simulink model "PID_uGrid_changed_by_code"  (R2020a)
settings: Solver=VariableStepAuto  StartTime=0.0  StopTime=0.08  RelTol=1e-3
values from neighbouring files (symbols this model uses):
  I_pv_sp_V = 0.0662*Ir_V+0.0549    [Simulation_PID_variable_conditions.m]    (also in Simulation_variable_PID_ANN_gain_selector.m; Simulation_variable_PID_Interpolated_gain_selector.m; Simulation_variable_PID_KNN_gain_selector.m)
  Ir_V = [0 100 500 1000 500 100 0]    [Simulation_PID_variable_conditions.m]    (also in Simulation_variable_PID_ANN_gain_selector.m; Simulation_variable_PID_Interpolated_gain_selector.m; Simulation_variable_PID_KNN_gain_selector.m)
  RL_var_vec = [1 6 8 15 7 3 5]    [Simulation_PID_variable_conditions.m]    (also in Simulation_variable_PID_ANN_gain_selector.m; Simulation_variable_PID_Interpolated_gain_selector.m; Simulation_variable_PID_KNN_gain_selector.m)
  tim_vec = 0:1:6    [Simulation_PID_variable_conditions.m]    (also in Simulation_variable_PID_ANN_gain_selector.m; Simulation_variable_PID_Interpolated_gain_selector.m; Simulation_variable_PID_KNN_gain_selector.m)
undefined symbols (not defined in the file or in its folder): fmicro, Ion, Lithium
libraries: powerlib x15, simulink x3, powerlib_meascontrol x3, eeStairGenerator x3, electricdrivelib x1, re_lib x1
settings Model: Creator=Javier  LastModifiedBy=Javier

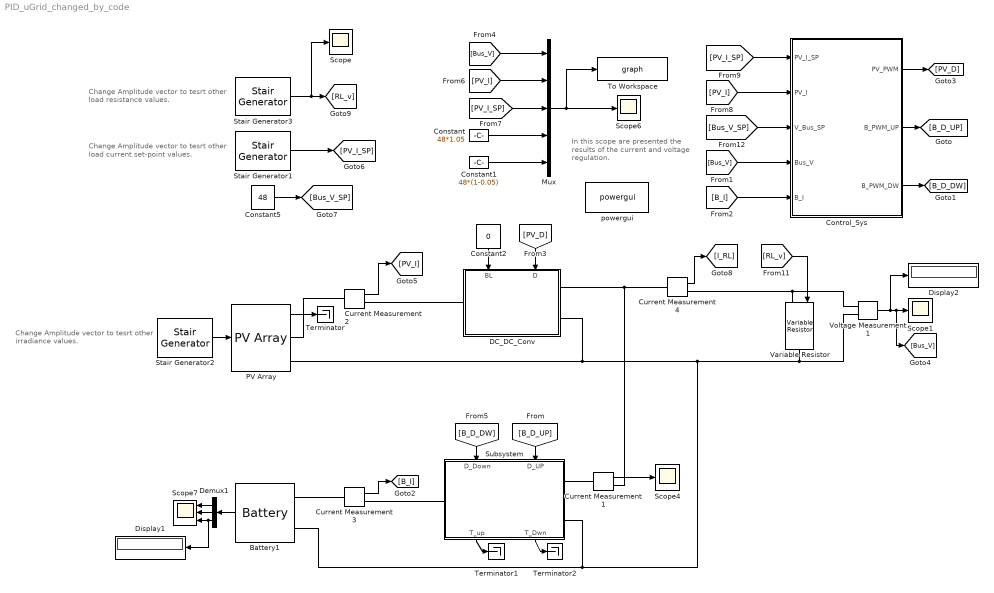
== system PID_uGrid_changed_by_code ==
  note: Change Amplitude vector to tesrt other
      | load resistance values.
  note: Change Amplitude vector to tesrt other
      | load current set-point values.
  note: Change Amplitude vector to tesrt other
      | irradiance values.
  note: In this scope are presented the
      | results of the current and voltage
      | regulation.
  Battery1 : electricdrivelib/Extra Sources/Battery  BatType=Lithium-Ion  ShowTempParam=off  ThermalPreset=no  ShowAgeParam=off  NomV=38.4  NomQ=2500  SOC=60  Batt_Tr=30  PresetModel=on  MaxQ=2500  MinV=28.8  FullV=44.6971  Dis_rate=1086.9565  R=0.0001536  Normal_OP=2260.8696  expZone="[41.48682      122.8261]"  current=[6.5 13 32.5]  Units=Time  Tci=20  NomT=20  T2=-30  MaxQ2=4.8  FullV2=7.1  Normal_OP2=5.655  expZone2="[6.58           1]"  Rca=0.6  ti=2000  Dp=0  Neq0=0  Tsim=1e6  Ta1=25  Qeol=5.4*0.9  Reol=0.013333*1.2  Char_age=[2.3478, 3]  Dis_age=[2.3478, 10]  N1=1500  N2=10500  N3=1000  N4=1400  Ta2=45  N5=950
  Constant : Constant  Value=48*1.05
  Constant1 : Constant  Value=48*(1-0.05)
  Constant2 : Constant  Value=0
  Constant5 : Constant  Value=48
  Control_Sys : Subsystem
  Current Measurement{1..4} (4 alike) : powerlib/Measurements/Current Measurement  PhasorSimulation=off  OutputType=Complex  PSBequivalent=0
  DC_DC_Conv : Subsystem
      settings: PortSchema="{\"entries\":[{\"content\":{\"sides\":[{\"content\":{\"connectorIds\":[\"LConn1\"]},\"type\":\"ConnectorPlacement.EquallySpacedRectSide\",\"uuid\":\"00f7090b-60ae-413e-b809-f771630d6751\"},{\"content\":{\"connectorIds\":[\"RConn1\",\"RConn2\"],\"side\":\"RIGHT\"},\"type\":\"ConnectorPlacement.EquallySpacedRectSide\",\"uuid\":\"f0025ab7-a9d8-466a-8e23-704d013948c1\"},{\"content\":{\"connectorIds\":[\"In1\",\"In2\"],\"side\":\"TOP\"},\"type\":\"ConnectorPlacement.EquallySpacedRectSide\",\"uuid\":\"5a345099-75bf-400d-9bb3-22f689fa92ef\"}]},\"type\":\"ConnectorPlacement.EquallySpacedConnector\",\"uuid\":\"2e1b2c5d-1adb-4779-83d3-3c40793dd951\"}],\"packageUris\":[\"http://schema.mathworks.com/mf0/Connector/19700101\"],\"version\":\"1.0\"}"
  Demux1 : Demux  Outputs=3
  Display1 : Display
  Display2 : Display
  Mux : Mux  Inputs=5
  PV Array : re_lib/Solar/PV Array  Npar=7  Nser=1  PlotType=array @ 1000 W/m2 & specified temperatures  S_vec="[ 1000  500  100 ]"  Temp_C_vec="[ 45 25  ]"  ModuleName=LG Electronics LG300N1W-G3  PlotWhenSelected=off  Pm=302.72  Ncell=60  Voc=39.5  Isc=10.05  Vm=32  Im=9.46  beta_Voc_pc=-0.3  alpha_Isc_pc=0.03  beta_Voc=-0.1185  alpha_Isc=0.003015  IL=10.0926  I0=3.3235e-11  nI=0.96984  Rsh=212.8143  Rs=0.31448  RobustModel=on  RobustCellTemperature=25  BAL=on  Tc=1e-7  Tfilter=1e-8
  Scope{,1,4,6} (4 alike) : Scope
  Scope7 : Scope  NumInputPorts=3
  Stair Generator1 : eeStairGenerator/Stair Generator  LabelModeActiveChoice=Discrete  TimeInput=[tim_vec]*0.01  AmplitudeInput=[I_pv_sp_V]  SampleTime=1/(1000e3)  RepeatPattern=off  OutDataTypeStr=double
      settings: SourceProductBaseCode=PS
  Stair Generator2 : eeStairGenerator/Stair Generator  LabelModeActiveChoice=Discrete  TimeInput=[tim_vec]*0.01  AmplitudeInput=[Ir_V]  SampleTime=1/(1000e3)  RepeatPattern=off  OutDataTypeStr=double
      settings: SourceProductBaseCode=PS
  Stair Generator3 : eeStairGenerator/Stair Generator  LabelModeActiveChoice=Discrete  TimeInput=[tim_vec]*0.01  AmplitudeInput=[RL_var_vec]  SampleTime=1/(1000e3)  RepeatPattern=off  OutDataTypeStr=double
      settings: SourceProductBaseCode=PS
  Subsystem : Subsystem
      settings: PortSchema="{\"entries\":[{\"content\":{\"sides\":[{\"content\":{\"connectorIds\":[\"LConn1\"]},\"type\":\"ConnectorPlacement.EquallySpacedRectSide\",\"uuid\":\"a9530ab3-8980-4dba-8483-d408c1c24a59\"},{\"content\":{\"connectorIds\":[\"RConn1\",\"RConn2\"],\"side\":\"RIGHT\"},\"type\":\"ConnectorPlacement.EquallySpacedRectSide\",\"uuid\":\"f691113d-6eb3-43ec-a6a4-3d8fb6884df6\"},{\"content\":{\"connectorIds\":[\"In1\",\"In2\"],\"side\":\"TOP\"},\"type\":\"ConnectorPlacement.EquallySpacedRectSide\",\"uuid\":\"a9eb11b6-05d7-4dbc-be9d-a17fd8550bb3\"},{\"content\":{\"connectorIds\":[\"Out1\",\"Out2\"],\"side\":\"BOTTOM\"},\"type\":\"ConnectorPlacement.EquallySpacedRectSide\",\"uuid\":\"90c7147c-e357-433a-9063-3b2a71587c45\"}]},\"type\":\"ConnectorPlacement.EquallySpacedConnector\",\"uuid\":\"b290d60f-d8ab-41f4-904b-2a909013e95d\"}],\"packageUris\":[\"http://schema.mathworks.com/mf0/Connector/19700101\"],\"version\":\"1.0\"}"
  Terminator : Terminator
  Terminator1 : Terminator
  Terminator2 : Terminator
  To Workspace : ToWorkspace  VariableName=graph  SaveFormat=Timeseries  SampleTime=-1
  Variable Resistor : powerlib/Elements/Variable Resistor  Rabsmin=1e-3
      settings: SourceProductBaseCode=PS
  Voltage Measurement1 : powerlib/Measurements/Voltage Measurement  PhasorSimulation=off  OutputType=Complex  PSBequivalent=0
  powergui : powerlib/powergui  Priority=1  SimulationMode=Discrete  SampleTime=1/(1000e3)  frequency=60  Iterations=50  frequencyindice=0  Pbase=100e6  ErrMax=1e-4  UnitsV=kV  UnitsW=MW  buscounter=0  FunctionMessages=off  echomessages=off  EnableUseOfTLC=off  CurrentSourceSwitches=off  DisableSnubberDevices=off  DisableRonSwitches=off  DisableVfSwitches=off  DisplayEquations=off  AutomaticDiscreteSolvers=off  SolverType=Tustin/Backward Euler (TBE)  Interpol=off  ExternalGateDelay=off  methode=off  Ts=100  x0status=blocks  SPID=on  SwTol=0  HookPort=off  NonlinearTolerance=1e-4  nMaxIteration=100  ContinueOnMaxIteration=off  RestoreLinks=warning  ResistiveCurrentMeasurement=off  Frange=[0:2:500]  Ylog=off  Xlog=on  ShowGrid=off  save=off  variable=ZData  structure=0  ZoomFFT=off  StartTime=0.0  cycles=1  DisplayStyle=1  fundamental=60  FreqAxis=off  MaxFrequency=1000  frequencyindicesteady=1  RmsSteady=1  display=off
  wires:
  Current Measurement1/1 -> Scope4/1
  Constant1/1 -> Mux/5
  Stair Generator2/1 -> PV Array/1
  Subsystem/1(T_up) -> Terminator1/1
  Subsystem/2(T_Dwn) -> Terminator2/1
  [B_D_UP] -> Subsystem/2(D_UP)
  [PV_I_SP] -> Control_Sys/1(PV_I_SP)
  [Bus_V] -> Mux/1
  [B_D_DW] -> Subsystem/1(D_Down)
  [PV_I] -> Control_Sys/2(PV_I)
  [Bus_V_SP] -> Control_Sys/3(V_Bus_SP)
  Constant5/1 -> [Bus_V_SP]
  Control_Sys/2(B_PWM_UP) -> [B_D_UP]
  [Bus_V] -> Control_Sys/4(Bus_V)
  PV Array/1 -> Terminator/1
  Current Measurement4/1 -> [I_RL]
  Battery1/1 -> Demux1/1
  Current Measurement3/1 -> [B_I]
  Constant2/1 -> DC_DC_Conv/1(BL)
  Control_Sys/3(B_PWM_DW) -> [B_D_DW]
  [PV_I] -> Mux/2
  Current Measurement2/1 -> [PV_I]
  Stair Generator3/1 -> Scope/1, [RL_v]
  Demux1/2 -> Scope7/2
  Control_Sys/1(PV_PWM) -> [PV_D]
  [B_I] -> Control_Sys/5(B_I)
  Voltage Measurement1/1 -> [Bus_V], Scope1/1, Display2/1
  [PV_I_SP] -> Mux/3
  Stair Generator1/1 -> [PV_I_SP]
  [RL_v] -> Variable Resistor/1
  Demux1/3 -> Display1/1, Scope7/3
  Demux1/1 -> Scope7/1
  Constant/1 -> Mux/4
  [PV_D] -> DC_DC_Conv/2(D)
  Mux/1 -> To Workspace/1, Scope6/1
  connections:
  DC_DC_Conv/RConn1 -- Current Measurement1/RConn1 -- Current Measurement4/LConn1
  Battery1/LConn2 -- Variable Resistor/RConn1 -- Voltage Measurement1/LConn2 -- DC_DC_Conv/RConn2 -- PV Array/RConn2 -- Subsystem/RConn2
  Voltage Measurement1/LConn1 -- Current Measurement4/RConn1 -- Variable Resistor/LConn1
  Current Measurement3/RConn1 -- Subsystem/LConn1
  Current Measurement2/RConn1 -- DC_DC_Conv/LConn1
  Current Measurement3/LConn1 -- Battery1/LConn1
  Current Measurement1/LConn1 -- Subsystem/RConn1
  Current Measurement2/LConn1 -- PV Array/RConn1

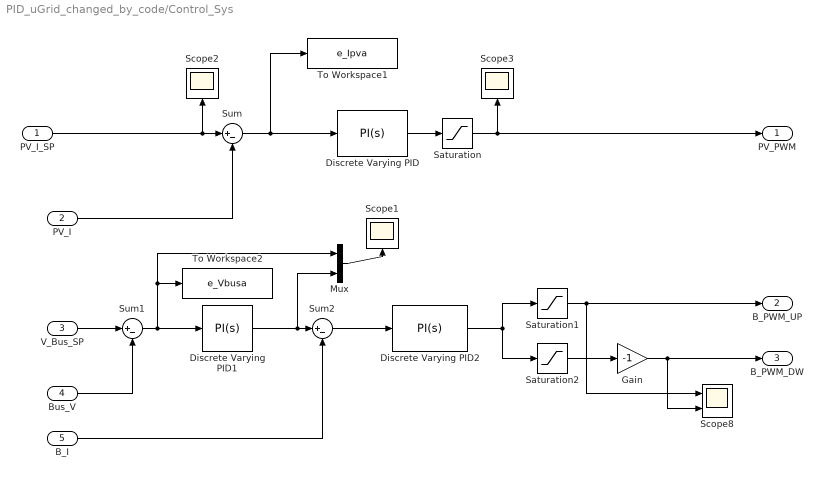
== system PID_uGrid_changed_by_code/Control_Sys ==
  PV_I_SP : Inport
  PV_I : Inport  Port=2
  V_Bus_SP : Inport  Port=3
  Bus_V : Inport  Port=4
  B_I : Inport  Port=5
  Discrete Varying PID : simulink/Continuous/PID Controller  Controller=PI  Form=Parallel  TimeDomain=Continuous-time  UseExternalTs=off  SampleTime=1/fmicro  IntegratorMethod=Forward Euler  FilterMethod=Forward Euler  ControllerParametersSource=internal  P=480.2696  I=467.6542  D=0  UseFilter=on  N=100  TunerSelectOption=Transfer Function Based (PID Tuner App)  InitialConditionSource=internal  InitialConditionForIntegrator=0  InitialConditionForFilter=0  DifferentiatorICPrevScaledInput=0  ExternalReset=none  TrackingMode=off  Kt=1  LimitOutput=on  UpperSaturationLimit=1  LowerSaturationLimit=-1  LinearizeAsGain=on  AntiWindupMode=none  Kb=1  POutMin=[]  POutMax=[]  IOutMin=[]  IOutMax=[]  DOutMin=[]  DOutMax=[]  NOutMin=[]  NOutMax=[]  SumOutMin=[]  SumOutMax=[]  SaturationOutMin=[]  SaturationOutMax=[]  PParamMin=[]  PParamMax=[]  IParamMin=[]  IParamMax=[]  DParamMin=[]  DParamMax=[]  NParamMin=[]  NParamMax=[]  KbParamMin=[]  KbParamMax=[]  KtParamMin=[]  KtParamMax=[]  KbOutMin=[]  KbOutMax=[]  KtOutMin=[]  KtOutMax=[]  IntegratorOutMin=[]  IntegratorOutMax=[]  FilterOutMin=[]  FilterOutMax=[]  SumI1OutMin=[]  SumI1OutMax=[]  SumI2OutMin=[]  SumI2OutMax=[]  SumI3OutMin=[]  SumI3OutMax=[]  SumI4OutMin=[]  SumI4OutMax=[]  SumDOutMin=[]  SumDOutMax=[]  DifferentiatorOutMin=[]  DifferentiatorOutMax=[]  FilterDiffOutCoefMin=[]  FilterDiffOutCoefMax=[]  ReciprocalOutMin=[]  ReciprocalOutMax=[]  SumDenOutMin=[]  SumDenOutMax=[]  SumNumOutMin=[]  SumNumOutMax=[]  DivideOutMin=[]  DivideOutMax=[]  UdiffTsProdOutMin=[]  UdiffTsProdOutMax=[]  NTsProdOutMin=[]  NTsProdOutMax=[]  UintegralTsProdOutMin=[]  UintegralTsProdOutMax=[]  UngainTsProdOutMin=[]  UngainTsProdOutMax=[]  IntegratorContinuousStateAttributes=''  IntegratorStateMustResolveToSignalObject=off  IntegratorRTWStateStorageClass=Auto  FilterContinuousStateAttributes=''  FilterStateMustResolveToSignalObject=off  FilterRTWStateStorageClass=Auto  ParallelPVariant=InternalParameters  IdealPVariant=Disabled  IVariant=InternalParameters  DVariant=Disabled  IntegratorVariant=Continuous  SatVariant=Enabled  AWVariant=Passthrough  PCopyVariant=Disabled  TRVariant=Disabled  FdbkBlocksVariant=Forward  IdealPFdbkVariant=Disabled  SatFdbkVariant=Disabled  DerivativeFilterVariant=Disabled  NVariant=Disabled  NCopyVariant=Disabled_SignalSpec  FilterICVariant=Disabled  IntegratorICVariant=InternalICs  ExternalResetVariant=Disabled  TRSumVariant=Passthrough  SumFdbkVariant=Disabled  SumVariant=Sum_PI  TsampFilterVariant=InternalTs  TsampNgainVariant=Passthrough  TsampIntegralVariant=Passthrough
  Discrete Varying PID1 : simulink/Continuous/PID Controller  Controller=PI  Form=Parallel  TimeDomain=Continuous-time  UseExternalTs=off  SampleTime=1/fmicro  IntegratorMethod=Forward Euler  FilterMethod=Forward Euler  ControllerParametersSource=internal  P=92.8314  I=4.166  D=0  UseFilter=on  N=100  TunerSelectOption=Transfer Function Based (PID Tuner App)  InitialConditionSource=internal  InitialConditionForIntegrator=0  InitialConditionForFilter=0  DifferentiatorICPrevScaledInput=0  ExternalReset=none  TrackingMode=off  Kt=1  LimitOutput=off  UpperSaturationLimit=500  LowerSaturationLimit=-500  LinearizeAsGain=on  AntiWindupMode=none  Kb=1  POutMin=[]  POutMax=[]  IOutMin=[]  IOutMax=[]  DOutMin=[]  DOutMax=[]  NOutMin=[]  NOutMax=[]  SumOutMin=[]  SumOutMax=[]  SaturationOutMin=[]  SaturationOutMax=[]  PParamMin=[]  PParamMax=[]  IParamMin=[]  IParamMax=[]  DParamMin=[]  DParamMax=[]  NParamMin=[]  NParamMax=[]  KbParamMin=[]  KbParamMax=[]  KtParamMin=[]  KtParamMax=[]  KbOutMin=[]  KbOutMax=[]  KtOutMin=[]  KtOutMax=[]  IntegratorOutMin=[]  IntegratorOutMax=[]  FilterOutMin=[]  FilterOutMax=[]  SumI1OutMin=[]  SumI1OutMax=[]  SumI2OutMin=[]  SumI2OutMax=[]  SumI3OutMin=[]  SumI3OutMax=[]  SumI4OutMin=[]  SumI4OutMax=[]  SumDOutMin=[]  SumDOutMax=[]  DifferentiatorOutMin=[]  DifferentiatorOutMax=[]  FilterDiffOutCoefMin=[]  FilterDiffOutCoefMax=[]  ReciprocalOutMin=[]  ReciprocalOutMax=[]  SumDenOutMin=[]  SumDenOutMax=[]  SumNumOutMin=[]  SumNumOutMax=[]  DivideOutMin=[]  DivideOutMax=[]  UdiffTsProdOutMin=[]  UdiffTsProdOutMax=[]  NTsProdOutMin=[]  NTsProdOutMax=[]  UintegralTsProdOutMin=[]  UintegralTsProdOutMax=[]  UngainTsProdOutMin=[]  UngainTsProdOutMax=[]  IntegratorContinuousStateAttributes=''  IntegratorStateMustResolveToSignalObject=off  IntegratorRTWStateStorageClass=Auto  FilterContinuousStateAttributes=''  FilterStateMustResolveToSignalObject=off  FilterRTWStateStorageClass=Auto  ParallelPVariant=InternalParameters  IdealPVariant=Disabled  IVariant=InternalParameters  DVariant=Disabled  IntegratorVariant=Continuous  SatVariant=Disabled  AWVariant=Passthrough  PCopyVariant=Disabled  TRVariant=Disabled  FdbkBlocksVariant=Forward  IdealPFdbkVariant=Disabled  SatFdbkVariant=Disabled  DerivativeFilterVariant=Disabled  NVariant=Disabled  NCopyVariant=Disabled_SignalSpec  FilterICVariant=Disabled  IntegratorICVariant=InternalICs  ExternalResetVariant=Disabled  TRSumVariant=Passthrough  SumFdbkVariant=Disabled  SumVariant=Sum_PI  TsampFilterVariant=InternalTs  TsampNgainVariant=Passthrough  TsampIntegralVariant=Passthrough
  Discrete Varying PID2 : simulink/Continuous/PID Controller  Controller=PI  Form=Parallel  TimeDomain=Continuous-time  UseExternalTs=off  SampleTime=1/fmicro  IntegratorMethod=Forward Euler  FilterMethod=Forward Euler  ControllerParametersSource=internal  P=0.01  I=36.8058  D=0  UseFilter=on  N=100  TunerSelectOption=Transfer Function Based (PID Tuner App)  InitialConditionSource=internal  InitialConditionForIntegrator=0  InitialConditionForFilter=0  DifferentiatorICPrevScaledInput=0  ExternalReset=none  TrackingMode=off  Kt=1  LimitOutput=on  UpperSaturationLimit=1  LowerSaturationLimit=-1  LinearizeAsGain=on  AntiWindupMode=none  Kb=1  POutMin=[]  POutMax=[]  IOutMin=[]  IOutMax=[]  DOutMin=[]  DOutMax=[]  NOutMin=[]  NOutMax=[]  SumOutMin=[]  SumOutMax=[]  SaturationOutMin=[]  SaturationOutMax=[]  PParamMin=[]  PParamMax=[]  IParamMin=[]  IParamMax=[]  DParamMin=[]  DParamMax=[]  NParamMin=[]  NParamMax=[]  KbParamMin=[]  KbParamMax=[]  KtParamMin=[]  KtParamMax=[]  KbOutMin=[]  KbOutMax=[]  KtOutMin=[]  KtOutMax=[]  IntegratorOutMin=[]  IntegratorOutMax=[]  FilterOutMin=[]  FilterOutMax=[]  SumI1OutMin=[]  SumI1OutMax=[]  SumI2OutMin=[]  SumI2OutMax=[]  SumI3OutMin=[]  SumI3OutMax=[]  SumI4OutMin=[]  SumI4OutMax=[]  SumDOutMin=[]  SumDOutMax=[]  DifferentiatorOutMin=[]  DifferentiatorOutMax=[]  FilterDiffOutCoefMin=[]  FilterDiffOutCoefMax=[]  ReciprocalOutMin=[]  ReciprocalOutMax=[]  SumDenOutMin=[]  SumDenOutMax=[]  SumNumOutMin=[]  SumNumOutMax=[]  DivideOutMin=[]  DivideOutMax=[]  UdiffTsProdOutMin=[]  UdiffTsProdOutMax=[]  NTsProdOutMin=[]  NTsProdOutMax=[]  UintegralTsProdOutMin=[]  UintegralTsProdOutMax=[]  UngainTsProdOutMin=[]  UngainTsProdOutMax=[]  IntegratorContinuousStateAttributes=''  IntegratorStateMustResolveToSignalObject=off  IntegratorRTWStateStorageClass=Auto  FilterContinuousStateAttributes=''  FilterStateMustResolveToSignalObject=off  FilterRTWStateStorageClass=Auto  ParallelPVariant=InternalParameters  IdealPVariant=Disabled  IVariant=InternalParameters  DVariant=Disabled  IntegratorVariant=Continuous  SatVariant=Enabled  AWVariant=Passthrough  PCopyVariant=Disabled  TRVariant=Disabled  FdbkBlocksVariant=Forward  IdealPFdbkVariant=Disabled  SatFdbkVariant=Disabled  DerivativeFilterVariant=Disabled  NVariant=Disabled  NCopyVariant=Disabled_SignalSpec  FilterICVariant=Disabled  IntegratorICVariant=InternalICs  ExternalResetVariant=Disabled  TRSumVariant=Passthrough  SumFdbkVariant=Disabled  SumVariant=Sum_PI  TsampFilterVariant=InternalTs  TsampNgainVariant=Passthrough  TsampIntegralVariant=Passthrough
  Gain : Gain  Gain=-1
  Mux : Mux  Inputs=2
  Saturation : Saturate  UpperLimit=1  LowerLimit=0
  Saturation1 : Saturate  UpperLimit=0.99  LowerLimit=0
  Saturation2 : Saturate  UpperLimit=0  LowerLimit=-0.99
  Scope1 : Scope
  Scope2 : Scope
  Scope3 : Scope
  Scope8 : Scope  NumInputPorts=2
  Sum : Sum  Inputs=|+-
  Sum1 : Sum  Inputs=|+-
  Sum2 : Sum  Inputs=|+-
  To Workspace1 : ToWorkspace  VariableName=e_Ipva  SaveFormat=Timeseries  SampleTime=-1
  To Workspace2 : ToWorkspace  VariableName=e_Vbusa  SaveFormat=Timeseries  SampleTime=-1
  PV_PWM : Outport
  B_PWM_UP : Outport  Port=2
  B_PWM_DW : Outport  Port=3
  wires:
  Saturation2/1 -> Gain/1
  PV_I/1 -> Sum/2
  Saturation/1 -> PV_PWM/1, Scope3/1
  Sum/1 -> Discrete Varying PID/1, To Workspace1/1
  Discrete Varying PID2/1 -> Saturation2/1, Saturation1/1
  Gain/1 -> B_PWM_DW/1, Scope8/2
  Saturation1/1 -> B_PWM_UP/1, Scope8/1
  B_I/1 -> Sum2/2
  Sum1/1 -> Mux/1, To Workspace2/1, Discrete Varying PID1/1
  V_Bus_SP/1 -> Sum1/1
  Bus_V/1 -> Sum1/2
  Discrete Varying PID/1 -> Saturation/1
  Discrete Varying PID1/1 -> Mux/2, Sum2/1
  Sum2/1 -> Discrete Varying PID2/1
  Mux/1 -> Scope1/1
  PV_I_SP/1 -> Scope2/1, Sum/1

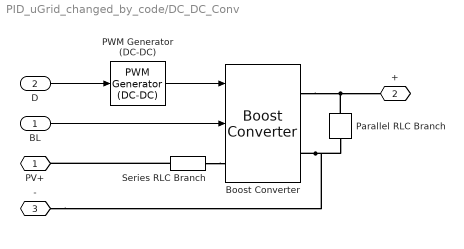
== system PID_uGrid_changed_by_code/DC_DC_Conv ==
  BL : Inport
  D : Inport  Port=2
  Boost Converter : powerlib/Power Electronics/Boost Converter  ModelType=Switching devices  Ron=1e-3  Rs=1e6  Cs=inf  Vforward=[0,0]  Ron_Diode=1e-3  Rs_Diode=1e6  Cs_Diode=inf  Vf_Diode=1e-3  Rs_CurrentSource=inf
      settings: SourceProductBaseCode=PS
  PWM Generator (DC-DC) : powerlib_meascontrol/Pulse & Signal Generators/PWM Generator (DC-DC)  Fsw=25e3  Ts=0
  Parallel RLC Branch : powerlib/Elements/Parallel RLC Branch  LConnTagsString=a  RConnTagsString=__new0  BranchType=C  Resistance=1e6  Inductance=1e-3  SetiL0=off  InitialCurrent=0  Capacitance=500e-6  Setx0=off  InitialVoltage=0  Measurements=None
  Series RLC Branch : powerlib/Elements/Series RLC Branch  LConnTagsString=__new0  RConnTagsString=__new0  BranchType=RL  Resistance=0.001  Inductance=96e-6  SetiL0=off  InitialCurrent=0  Capacitance=1e-6  Setx0=off  InitialVoltage=0  Measurements=None
  PV+ : PMIOPort  Side=Left
  + : PMIOPort  Port=2  Side=Right
  - : PMIOPort  Port=3  Side=Right
  wires:
  D/1 -> PWM Generator (DC-DC)/1
  PWM Generator (DC-DC)/1 -> Boost Converter/1
  BL/1 -> Boost Converter/2
  connections:
  Series RLC Branch/LConn1 -- PV+/RConn1
  Parallel RLC Branch/LConn1 -- Boost Converter/RConn1 -- +/RConn1
  Series RLC Branch/RConn1 -- Boost Converter/LConn1
  Boost Converter/RConn2 -- -/RConn1 -- Parallel RLC Branch/RConn1

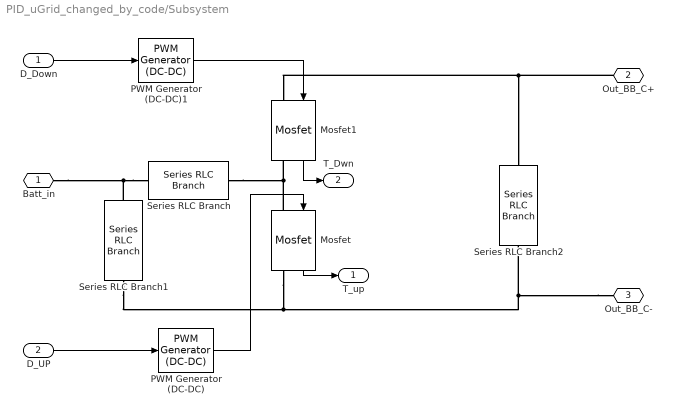
== system PID_uGrid_changed_by_code/Subsystem ==
  D_Down : Inport
  D_UP : Inport  Port=2
  Mosfet : powerlib/Power Electronics/Mosfet  Ron=0.1  Lon=0  Rd=0.01  Vfd=0  IC=0  Rs=1e5  Cs=inf  Measurements=on
  Mosfet1 : powerlib/Power Electronics/Mosfet  Ron=0.1  Lon=0  Rd=0.01  Vfd=0  IC=0  Rs=1e5  Cs=inf  Measurements=on
  PWM Generator (DC-DC) : powerlib_meascontrol/Pulse & Signal Generators/PWM Generator (DC-DC)  Fsw=25e3  Ts=0
  PWM Generator (DC-DC)1 : powerlib_meascontrol/Pulse & Signal Generators/PWM Generator (DC-DC)  Fsw=25e3  Ts=0
  Series RLC Branch : powerlib/Elements/Series RLC Branch  LConnTagsString=__new0  RConnTagsString=__new0  BranchType=L  Resistance=1  Inductance=5e-6  SetiL0=off  InitialCurrent=0  Capacitance=1e-6  Setx0=off  InitialVoltage=0  Measurements=None
  Series RLC Branch1 : powerlib/Elements/Series RLC Branch  LConnTagsString=__new0  RConnTagsString=__new0  BranchType=RC  Resistance=1  Inductance=1e-3  SetiL0=off  InitialCurrent=0  Capacitance=48e-6  Setx0=off  InitialVoltage=0  Measurements=None
  Series RLC Branch2 : powerlib/Elements/Series RLC Branch  LConnTagsString=__new0  RConnTagsString=__new0  BranchType=C  Resistance=1  Inductance=1e-3  SetiL0=off  InitialCurrent=0  Capacitance=48e-6  Setx0=off  InitialVoltage=0  Measurements=None
  Batt_in : PMIOPort  Side=Left
  Out_BB_C+ : PMIOPort  Port=2  Side=Right
  Out_BB_C- : PMIOPort  Port=3  Side=Right
  T_up : Outport
  T_Dwn : Outport  Port=2
  wires:
  PWM Generator (DC-DC)/1 -> Mosfet/1
  PWM Generator (DC-DC)1/1 -> Mosfet1/1
  Mosfet/1 -> T_up/1
  D_Down/1 -> PWM Generator (DC-DC)1/1
  Mosfet1/1 -> T_Dwn/1
  D_UP/1 -> PWM Generator (DC-DC)/1
  connections:
  Out_BB_C-/RConn1 -- Series RLC Branch2/RConn1 -- Mosfet/RConn1 -- Series RLC Branch1/RConn1
  Series RLC Branch/LConn1 -- Batt_in/RConn1 -- Series RLC Branch1/LConn1
  Out_BB_C+/RConn1 -- Mosfet1/LConn1 -- Series RLC Branch2/LConn1
  Mosfet/LConn1 -- Series RLC Branch/RConn1 -- Mosfet1/RConn1
